simulink subsystem "State_Interpreter"  (R2023b)
settings: Solver=VariableStepAuto  StartTime=0.0  StopTime=10.0  RelTol=1e-3
undefined symbols (not defined in the file): data, InstantState, t_sample
libraries: simulink x3
settings Model: Creator=FIRSTMentor  LastModifiedBy=FIRSTMentor

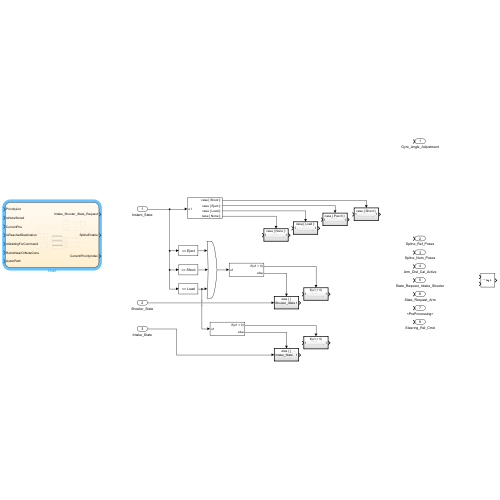
[thumbnail: Simulink's stored preview of the top-level diagram]
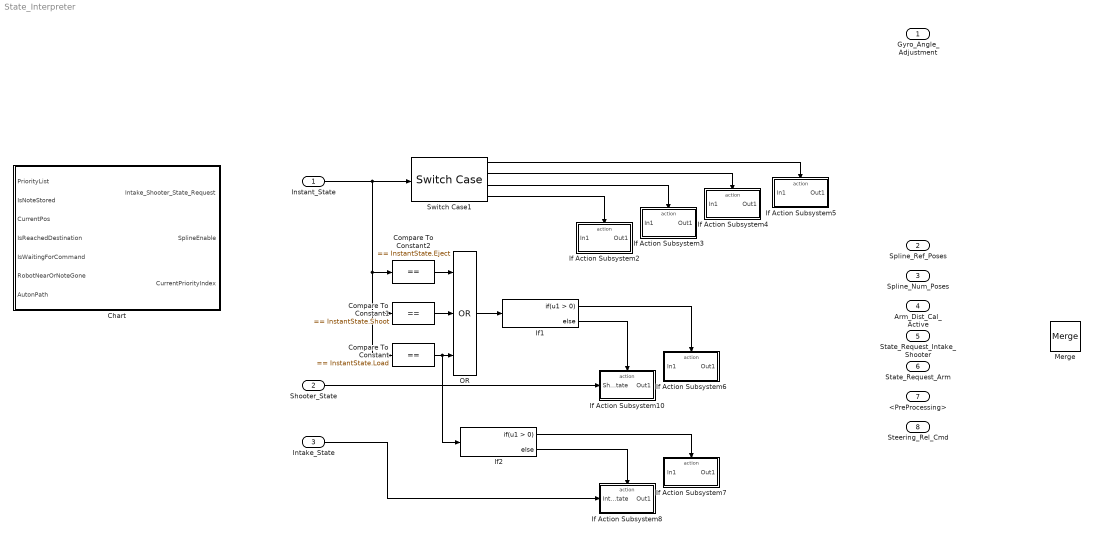
== system State_Interpreter ==
  Instant_State : Inport  OutDataTypeStr=Enum: InstantState
  Shooter_State : Inport  Port=2  OutDataTypeStr=Enum: ShooterState
  Intake_State : Inport  Port=3  OutDataTypeStr=Enum: IntakeState
  Chart : Stateflow chart  TreatAsAtomicUnit=on
  Compare To Constant : simulink/Logic and Bit Operations/Compare To Constant  relop===  const=InstantState.Load  OutDataTypeStr=boolean
  Compare To Constant1 : simulink/Logic and Bit Operations/Compare To Constant  relop===  const=InstantState.Shoot  OutDataTypeStr=boolean
  Compare To Constant2 : simulink/Logic and Bit Operations/Compare To Constant  relop===  const=InstantState.Eject  OutDataTypeStr=boolean
  If Action Subsystem10 : Subsystem  TreatAsAtomicUnit=on
  If Action Subsystem2 : Subsystem  TreatAsAtomicUnit=on
  If Action Subsystem3 : Subsystem  TreatAsAtomicUnit=on
  If Action Subsystem4 : Subsystem  TreatAsAtomicUnit=on
  If Action Subsystem5 : Subsystem  TreatAsAtomicUnit=on
  If Action Subsystem6 : Subsystem  TreatAsAtomicUnit=on
  If Action Subsystem7 : Subsystem  TreatAsAtomicUnit=on
  If Action Subsystem8 : Subsystem  TreatAsAtomicUnit=on
  If1 : If
  If2 : If
  Merge : Merge
  OR : Logic  Operator=OR  Inputs=3  IconShape=distinctive  AllPortsSameDT=off  OutDataTypeStr=boolean
  Switch Case1 : SwitchCase  CaseConditions={InstantState.Shoot, InstantState.Eject, InstantState.Load, InstantState.None}  ShowDefaultCase=off
  Gyro_Angle_Adjustment : Outport
  Spline_Ref_Poses : Outport  Port=2
  Spline_Num_Poses : Outport  Port=3
  Arm_Dist_Cal_Active : Outport  Port=4
  State_Request_Intake_Shooter : Outport  Port=5
  State_Request_Arm : Outport  Port=6
  <PreProcessing> : Outport  Port=7
  Steering_Rel_Cmd : Outport  Port=8
  wires:
  Switch Case1/1 -> If Action Subsystem5/Action
  Switch Case1/2 -> If Action Subsystem4/Action
  Switch Case1/3 -> If Action Subsystem3/Action
  Switch Case1/4 -> If Action Subsystem2/Action
  Compare To Constant/1 -> If2/1, OR/3
  Compare To Constant2/1 -> OR/1
  Compare To Constant1/1 -> OR/2
  OR/1 -> If1/1
  Instant_State/1 -> Switch Case1/1, Compare To Constant/1, Compare To Constant1/1, Compare To Constant2/1
  If1/2 -> If Action Subsystem10/Action
  If1/1 -> If Action Subsystem6/Action
  Shooter_State/1 -> If Action Subsystem10/1(Shooter_State)
  Intake_State/1 -> If Action Subsystem8/1(Intake_State)
  If2/1 -> If Action Subsystem7/Action
  If2/2 -> If Action Subsystem8/Action

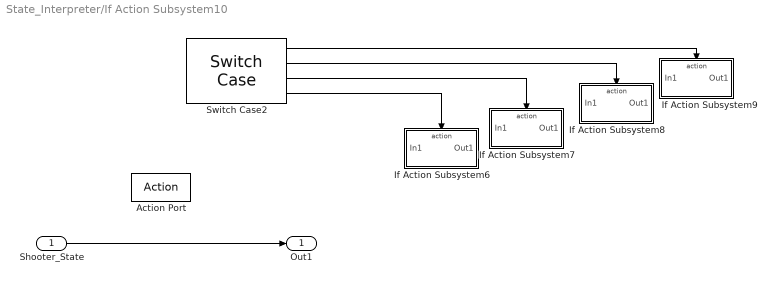
== system State_Interpreter/If Action Subsystem10 ==
  Shooter_State : Inport
  Action Port : ActionPort  ActionPortLabel=else
  If Action Subsystem6 : Subsystem  TreatAsAtomicUnit=on
  If Action Subsystem7 : Subsystem  TreatAsAtomicUnit=on
  If Action Subsystem8 : Subsystem  TreatAsAtomicUnit=on
  If Action Subsystem9 : Subsystem  TreatAsAtomicUnit=on
  Switch Case2 : SwitchCase  CaseConditions={ShooterState.Trap, ShooterState.Amp, ShooterState.Angle, ShooterState.Home}  ShowDefaultCase=off
  Out1 : Outport
  wires:
  Shooter_State/1 -> Out1/1
  Switch Case2/1 -> If Action Subsystem9/Action
  Switch Case2/3 -> If Action Subsystem7/Action
  Switch Case2/2 -> If Action Subsystem8/Action
  Switch Case2/4 -> If Action Subsystem6/Action

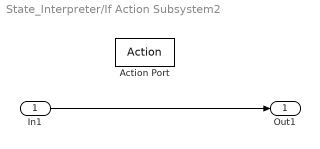
== system State_Interpreter/If Action Subsystem2 ==
  In1 : Inport
  Action Port : ActionPort  ActionPortLabel=case [ None ]:
  Out1 : Outport
  wires:
  In1/1 -> Out1/1

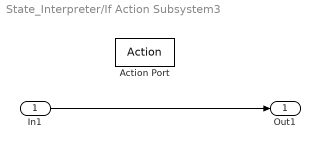
== system State_Interpreter/If Action Subsystem3 ==
  In1 : Inport
  Action Port : ActionPort  ActionPortLabel=case [ Load ]:
  Out1 : Outport
  wires:
  In1/1 -> Out1/1

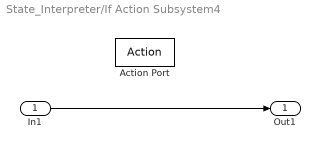
== system State_Interpreter/If Action Subsystem4 ==
  In1 : Inport
  Action Port : ActionPort  ActionPortLabel=case [ Pooch ]:
  Out1 : Outport
  wires:
  In1/1 -> Out1/1

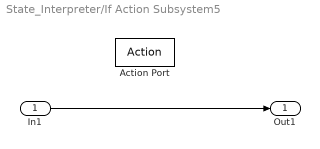
== system State_Interpreter/If Action Subsystem5 ==
  In1 : Inport
  Action Port : ActionPort  ActionPortLabel=case [ Shoot ]:
  Out1 : Outport
  wires:
  In1/1 -> Out1/1

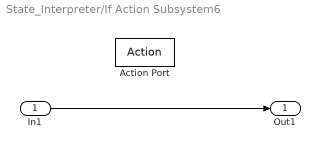
== system State_Interpreter/If Action Subsystem6 ==
  In1 : Inport
  Action Port : ActionPort  ActionPortLabel=if(u1 > 0)
  Out1 : Outport
  wires:
  In1/1 -> Out1/1

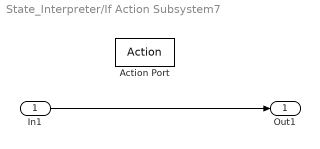
== system State_Interpreter/If Action Subsystem7 ==
  In1 : Inport
  Action Port : ActionPort  ActionPortLabel=if(u1 > 0)
  Out1 : Outport
  wires:
  In1/1 -> Out1/1

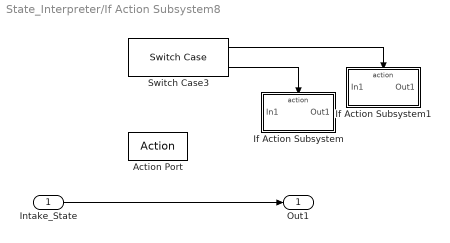
== system State_Interpreter/If Action Subsystem8 ==
  Intake_State : Inport
  Action Port : ActionPort  ActionPortLabel=else
  If Action Subsystem : Subsystem  TreatAsAtomicUnit=on
  If Action Subsystem1 : Subsystem  TreatAsAtomicUnit=on
  Switch Case3 : SwitchCase  CaseConditions={IntakeState.On, IntakeState.Off}  ShowDefaultCase=off
  Out1 : Outport
  wires:
  Intake_State/1 -> Out1/1
  Switch Case3/1 -> If Action Subsystem1/Action
  Switch Case3/2 -> If Action Subsystem/Action

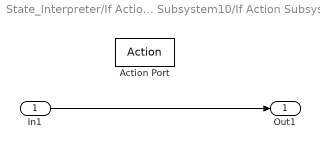
== system State_Interpreter/If Action Subsystem10/If Action Subsystem6 ==
  In1 : Inport
  Action Port : ActionPort  ActionPortLabel=case [ Home ]:
  Out1 : Outport
  wires:
  In1/1 -> Out1/1

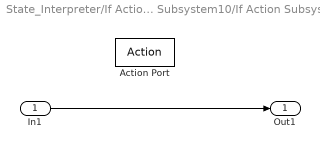
== system State_Interpreter/If Action Subsystem10/If Action Subsystem7 ==
  In1 : Inport
  Action Port : ActionPort  ActionPortLabel=case [ Angle ]:
  Out1 : Outport
  wires:
  In1/1 -> Out1/1

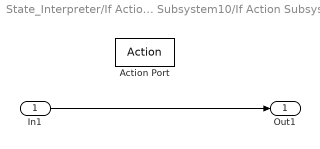
== system State_Interpreter/If Action Subsystem10/If Action Subsystem8 ==
  In1 : Inport
  Action Port : ActionPort  ActionPortLabel=case [ Amp ]:
  Out1 : Outport
  wires:
  In1/1 -> Out1/1

== system State_Interpreter/If Action Subsystem10/If Action Subsystem9 ==
  In1 : Inport
  Action Port : ActionPort  ActionPortLabel=case [ Trap ]:
  Out1 : Outport
  wires:
  In1/1 -> Out1/1

== system State_Interpreter/If Action Subsystem8/If Action Subsystem ==
  In1 : Inport
  Action Port : ActionPort  ActionPortLabel=case [ Off ]:
  Out1 : Outport
  wires:
  In1/1 -> Out1/1

== system State_Interpreter/If Action Subsystem8/If Action Subsystem1 ==
  In1 : Inport
  Action Port : ActionPort  ActionPortLabel=case [ On ]:
  Out1 : Outport
  wires:
  In1/1 -> Out1/1

== stateflow chart State_Interpreter/Chart ==
  state CheckForRobotOrNoteWODetec
    en:
    Intake_Shooter_State_Request = 0;
    Timer = t_sample;
    du:
    Timer = Timer + t_sample;
    ex:
    CurrentPriorityIndex = CurrentPriorityIndex + 1;
  state ShootWODetec
    en:
    Intake_Shooter_State_Request = 1;
    Timer = t_sample;
    du:
    Timer = Timer + t_sample;
    ex:
    Intake_Shooter_State_Request = 0;
  state PathToPickUpWODetec
    en:
    SplineEnable = 1;
    ex:
    SplineEnable = 0;
  state RunIntakeWODetec
    en:
    SplineEnable = 1;
    Intake_Shooter_State_Request = 1;
    Timer = t_sample;
    du:
    Timer = Timer + t_sample;
    ex:
    Intake_Shooter_State_Request = 0;
    SplineEnable = 0;
  state PathToShootWODetec
    en:
    SplineEnable = 1;
    ex:
    SplineEnable = 0;
  state PathPicker
    en:
    CloseNoteCounter = 0;
  state Auto Detection [group]
    path will be path
    10
  state CheckForRobotOrNote
    en:
    Intake_Shooter_State_Request = 0;
    SplineEnable = 0;
    Timer = t_sample;
    du:
    Timer = Timer + t_sample;
    ex:
    CurrentPriorityIndex = CurrentPriorityIndex + 1;
  state Note6
    state Shoot1
      en:
      Intake_Shooter_State_Request = 1;
      SplineEnable = 0;
      Timer = t_sample;
      du:
      Timer = Timer + t_sample;
      ex:
      Intake_Shooter_State_Request = 0;
    state PathToShoot1
      en:
      SplineEnable = 1;
      CloseNoteCounter = CloseNoteCounter + 1;
      ex:
      SplineEnable = 0;
    174 -> Note6.PathToShoot1
    Note6.PathToShoot1 -> Note6.Shoot1
    Note6.Shoot1 -> 179 : [IsWaitingForCommand]
  state Shoot
    en:
    Intake_Shooter_State_Request = 1;
    SplineEnable = 0;
    Timer = t_sample;
    du:
    Timer = Timer + t_sample;
    ex:
    Intake_Shooter_State_Request = 0;
  state PathToPickUp
    en:
    SplineEnable = 1;
    ex:
    SplineEnable = 0;
  state Note6_trans
  state Note7
    state Shoot1
      en:
      Intake_Shooter_State_Request = 1;
      SplineEnable = 0;
      Timer = t_sample;
      du:
      Timer = Timer + t_sample;
      ex:
      Intake_Shooter_State_Request = 0;
    state PathToShoot1
      en:
      SplineEnable = 1;
      CloseNoteCounter = CloseNoteCounter + 1;
      ex:
      SplineEnable = 0;
    Note7.Shoot1 -> 186 : [IsWaitingForCommand]
    187 -> Note7.PathToShoot1
    Note7.PathToShoot1 -> Note7.Shoot1
  state Note7_trans
  state End
  state RunIntake
    en:
    SplineEnable = 1;
    Intake_Shooter_State_Request = 1;
    ex:
    Intake_Shooter_State_Request = 0;
    SplineEnable = 0;
  state PathToShoot
    en:
    SplineEnable = 1;
    ex:
    SplineEnable = 0;
  state Note8
    state Shoot1
      en:
      Intake_Shooter_State_Request = 1;
      SplineEnable = 0;
      Timer = t_sample;
      du:
      Timer = Timer + t_sample;
      ex:
      Intake_Shooter_State_Request = 0;
    state PathToShoot1
      en:
      SplineEnable = 1;
      CloseNoteCounter = CloseNoteCounter + 1;
      ex:
      SplineEnable = 0;
    197 -> Note8.PathToShoot1
    Note8.PathToShoot1 -> Note8.Shoot1
    Note8.Shoot1 -> 196 : [IsWaitingForCommand]
  state Note8_trans
  ShootWODetec -> PathToPickUpWODetec : [IsWaitingForCommand || Timer > 16]
  PathToPickUpWODetec -> CheckForRobotOrNoteWODetec : [IsReachedDestination]
  (junction 524) -> PathToPickUpWODetec
  CheckForRobotOrNoteWODetec -> RunIntakeWODetec : [IsWaitingForCommand || Timer >= 16]
  PathToShootWODetec -> ShootWODetec [order 2] : [IsReachedDestination]
  (junction 522) -> (junction 524)
  (junction 515) -> (junction 517)
  (junction 482) -> (junction 524)
  (junction 517) -> (junction 518)
  PathPicker -> (junction 522) [order 5]
  PathToShootWODetec -> (junction 515) [order 1] : [PriorityList(CurrentPriorityIndex) == null]
  RunIntakeWODetec -> PathToShootWODetec : [IsNoteStored || Timer >= 16]
  (default) -> PathPicker
  PathPicker -> (junction 423) [order 4] : [AutonPath == 3]
  (junction 423) -> (junction 216)
  PathPicker -> (junction 422) [order 3] : [AutonPath == 2]
  (junction 422) -> (junction 214)
  PathPicker -> (junction 267) [order 2] : [AutonPath == 1]
  (junction 267) -> (junction 212)
  PathPicker -> Shoot [order 1] : [AutonPath == 10]
  (junction 428) -> (junction 482)
  Shoot -> PathToPickUp [order 1] : [PriorityList(CurrentPriorityIndex) < 6]
  PathToPickUp -> CheckForRobotOrNote [order 1] : [Timer  < 16]
  180 -> Note6_trans
  Note6_trans -> (junction 125) [order 5] : [~IsWaitingForCommand]
  CheckForRobotOrNote -> PathToPickUp [order 3] : [PriorityList(CurrentPriorityIndex) < 6 && RobotNearOrNoteGone]
  (junction 90) -> (junction 212)
  (junction 212) -> 175
  (junction 125) -> End
  (junction 229) -> (junction 212)
  (junction 89) -> (junction 90) [order 1] : [PriorityList(CurrentPriorityIndex) == 6 || (CurrentPos == (1) || (2))]
  Note6_trans -> (junction 428) [order 4] : [CloseNoteCounter == 3 && ( AutonPath == 3 || AutonPath == 2)]
  Note6_trans -> (junction 220) [order 3] : [~IsReachedDestination]
  Note7_trans -> Note6_trans [order 2] : [CloseNoteCounter == 2]
  Note6_trans -> Note7_trans [order 2] : [CloseNoteCounter == 1]
  Note8_trans -> Note6_trans [order 2] : [CloseNoteCounter == 2]
  Note6_trans -> Note8_trans [order 1] : [CloseNoteCounter == 2]
  (junction 430) -> (junction 428)
  PathToPickUp -> (junction 50) [order 2] : [Timer  < 16]
  CheckForRobotOrNote -> (junction 49) [order 2] : [PriorityList(CurrentPriorityIndex) > 5 && RobotNearOrNoteGone]
  CheckForRobotOrNote -> RunIntake [order 1] : [~RobotNearOrNoteGone]
  (junction 220) -> (junction 229)
  PathToShoot -> Shoot [order 1] : [PriorityList(CurrentPriorityIndex) < 6]
  Shoot -> (junction 51) [order 2] : [PriorityList(CurrentPriorityIndex) > 5]
  (junction 518) -> End
  184 -> Note7_trans
  Note7_trans -> End [order 4] : [~IsWaitingForCommand]
  (junction 89) -> (junction 214) [order 3] : [PriorityList(CurrentPriorityIndex) == 7 || CurrentPos == 3]
  (junction 214) -> 183
  (junction 51) -> (junction 89)
  (junction 49) -> (junction 50) : [Timer  < 16]
  (junction 50) -> (junction 51)
  (junction 89) -> (junction 92) [order 2] : [PriorityList(CurrentPriorityIndex) == 8 || (CurrentPos == (4) || (5) )]
  (junction 226) -> (junction 214)
  RunIntake -> (junction 49) [order 2] : [~IsNoteStored &&PriorityList(CurrentPriorityIndex) < 6 ]
  PathToShoot -> (junction 51) [order 2] : [PriorityList(CurrentPriorityIndex) > 5]
  Note7_trans -> (junction 221) [order 3] : [~IsReachedDestination]
  Note8_trans -> Note7_trans [order 1] : [CloseNoteCounter == 1]
  Note7_trans -> Note8_trans [order 1] : [CloseNoteCounter == 1]
  (junction 128) -> End
  (junction 221) -> (junction 226)
  RunIntake -> PathToShoot [order 1] : [IsNoteStored]
  194 -> Note8_trans
  Note8_trans -> (junction 128) [order 5] : [~IsWaitingForCommand]
  (junction 92) -> (junction 216)
  (junction 216) -> 193
  (junction 223) -> (junction 216)
  Note8_trans -> (junction 430) [order 4] : [CloseNoteCounter == 3 && AutonPath == 1]
  Note8_trans -> (junction 222) [order 3] : [~IsReachedDestination]
  (junction 222) -> (junction 223)
  data: PriorityList input; Intake_Shooter_State_Request output; IsNoteStored input; CurrentPos input; SplineEnable output; IsReachedDestination input; CurrentPriorityIndex output =1; Timer local; t_sample parameter; IsWaitingForCommand input; RobotNearOrNoteGone input; CloseNoteCounter local; AutonPath input; data parameter
